simulink model "sphere_position_model"  (R2021b)
settings: Solver=FixedStepAuto  StartTime=0.0  StopTime=10.0  FixedStep=0.1  RelTol=1e-3
undefined symbols (not defined in the file): masseSeff
settings Model: Creator=dupa1607  LastModifiedBy=alexi
settings SolverCC: AlgebraicLoopSolver=TrustRegion
settings DebuggingCC: SFMachineParentedDataDiag=warning

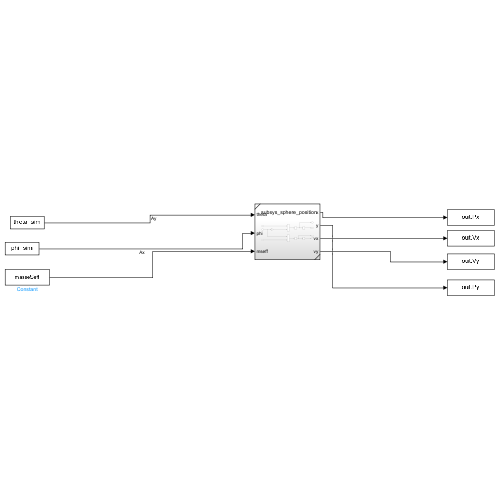
[thumbnail: Simulink's stored preview of the top-level diagram]
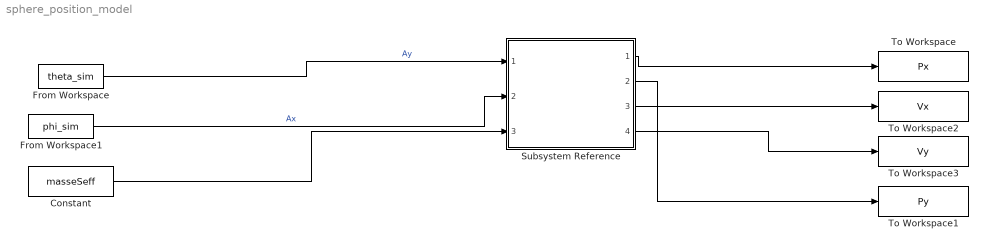
== system sphere_position_model ==
  Constant : Constant  Value=masseSeff
  From Workspace : FromWorkspace  VariableName=theta_sim
  From Workspace1 : FromWorkspace  VariableName=phi_sim
  Subsystem Reference : Subsystem  ReferencedSubsystem=subsys_sphere_position
  To Workspace : ToWorkspace  VariableName=Px  SaveFormat=Timeseries  SampleTime=-1
  To Workspace1 : ToWorkspace  VariableName=Py  SaveFormat=Timeseries  SampleTime=-1
  To Workspace2 : ToWorkspace  VariableName=Vx  SaveFormat=Timeseries  SampleTime=-1
  To Workspace3 : ToWorkspace  VariableName=Vy  SaveFormat=Timeseries  SampleTime=-1
  wires:
  From Workspace/1 -> Subsystem Reference/1  "Ay"
  From Workspace1/1 -> Subsystem Reference/2  "Ax"
  Subsystem Reference/1 -> To Workspace/1
  Subsystem Reference/2 -> To Workspace1/1
  Constant/1 -> Subsystem Reference/3
  Subsystem Reference/3 -> To Workspace2/1
  Subsystem Reference/4 -> To Workspace3/1
